simulink model "ModelGridFormingController"  (R2025b)
settings: Solver=ode1be  StartTime=0.0  StopTime=6  FixedStep=gridInverter.vsm.samplingTime  MaxStep=gridInverter.vsm.samplingTime  RelTol=1e-3  AbsTol=1e-3
PreLoadFcn:
  | % Parameterize the model
  | TestGridFormingControllerInputParameters;
values from neighbouring files (symbols this model uses):
  localSolverSampleTime = 100e-6    (= 0.0001)    [TestGridFormingControllerInputParameters.m]
undefined symbols (not defined in the file or in its folder): base, gridInverter
libraries: ee_lib x8, nesl_utility x5, fl_lib x3, eeGeneralControl x2, eeSinGeneratorThreePhase x1, GFMLibrary x1
CloseFcn:
  | try, close( 'GridFormingConverterNormalOperation'), end
  | try, close( 'GridFormingConverterActivePowerChange'), end
  | try, close( 'GridFormingConverterReactivePowerChange'), end
  | try, close( 'GridFormingConverterGridVoltageChange'), end
  | try, close( 'GridFormingConverterLocalLoadChange'), end
  | try, close( 'GridFormingConverterSmallGridFreqChange'), end
  | try, close( 'GridFormingConverterLargeGridFreqChange'), end
  | try, close( 'GridFormingConverterFullGridFreqChange'), end
  | try, close( 'GridFormingConverter10DegGridPhaseChange'), end
  | try, close( 'GridFormingConverter60DegGridPhaseChange'), end
  | try, close( 'GridFormingConverterPermanentFault'), end
  | try, close( 'GridFormingConverterTemporaryFault'), end
  | try, close( 'GridFormingConverterActivePowerChangeWithRipple'), end
  | try, close( 'GridFormingConverterIslanding'), end
  | try, close( 'GridFormingConverterDampingEffect'), end
  | try, close( 'GridFormingConverterIntertiaEffect'), end
  | try, close('GridFormingConverterVdControllerBodePlot'), end
  | try, close('GridFormingConverterControllerBodePlot'), end
  | try, close( 'GridFormingConverterThreePhaseFault'), end
  | try, close( 'GridFormingConverterThreePhaseFaultStandard'), end
  | try, close( 'GridFormingConverterCompareFaultRideMethod'), end
  | clear base currentLimitMethodSelected expectedSCR
  | clear grid gridInverter primaryBaseImpedance
  | clear realPowerMethodSelected scrSelected scrFactor
  | clear seconadryBaseImpedance shortCircuit
  | clear simulationTime systemSCR testConditionSelected
  | clear testCondition tout transformer TransmissionLine
  | clear gridVoltageProfileVal gridVoltageProfileTime
  | clear gridFrequencyProfileVal gridFrequencyProfileTime
  | clear gridVoltageProfileVal gridVoltageProfileTime
  | clear gridFrequencyProfileVal gridFrequencyProfileTime
  | clear gridPhaseProfileVal gridPhaseProfileTime
  | clear gfmRealPowerRefProfileVal gfmRealPowerRefProfileTime
  | clear gfmControllerRippleInjectMagVal gfmControllerRippleInjectMagTime
  | clear gfmControllerRippleInjectFreqVal gfmControllerRippleInjectFreqTime
  | clear gfmReactivePowerRefProfileVal gfmReactivePowerRefProfileTime
  | clear localLoadRealProfileVal localLoadRealProfileTime
  | clear localLoadReactiveProfileVal localLoadReactiveProfileTime
  | clear faultTriggerVal faultTriggerTime
  | clear circuitBreakerTripSignalVal circuitBreakerTripSignalTime
  | clear disturbanceTime realPartImpedance  localSolverSampleTime
  | clear SimlogGridFormingConverter temprySampleData
  | clear outValue outputTable plotFlag margintable testOutcome
  | clear realPart  XbyRtempFactor scrFactorXg scrFactorRg scrOut XbyROut systemSCR
  | clear outTable marginTable controllerName dampingArray inertiaConstantArray
  | clear imaginaryPart LogsoutGridFormingConverter faultImpedanceArray
  | clear outData
Description:
  | Design and Analysis of Grid-Forming Converter
settings Model: ExtModeTrigDuration=100  Creator=The MathWorks, Inc.  LastModifiedBy=vsolaise
settings SolverCC: AutoScaleAbsTol=off  AlgebraicLoopSolver=TrustRegion
settings DataIOCC: SaveOutput=off  DSMLogging=off  StateSaveName=tmp_raccel_xout  SignalLoggingName=LogsoutGridFormingConverter  OutputTimes=[0:1.1*3*Voc/(1*2000):1.1*3*Voc/1]  ReturnWorkspaceOutputsName=outData
settings OptimizationCC: ReuseModelBlockBuffer=off  EfficientMapNaN2IntZero=off
settings DebuggingCC: AlgebraicLoopMsg=none  StateNameClashWarn=warning  ArithmeticOperatorsInVariantConditions=warning
settings HardwareCC: ProdBitPerPointer=32.0  ProdBitPerSizeT=32.0  ProdBitPerPtrDiffT=32.0  ProdWordSize=32.0  ProdHWDeviceType=Intel->x86-32 (Windows32)  TargetBitPerPointer=64.0  TargetBitPerSizeT=64.0  TargetBitPerPtrDiffT=64.0  TargetLongLongMode=on  TargetIntDivRoundTo=Zero  TargetEndianess=LittleEndian  TargetWordSize=64.0  TargetHWDeviceType=MATLAB Host  ProdEqTarget=off
settings ModelReferenceCC: EnableRefExpFcnMdlSchedulingChecks=on  PropagateSignalLabelsOutOfModel=off
settings SFSimCC: CustomCodeUndefinedFunction=UseInterfaceOnly
settings RTWCC: SystemTargetFile=raccel.tlc  TemplateMakefile=raccel_default_tmf  RTWVerbose=off  RTWUseSimCustomCode=on  GPUComputeCapability=3.5
settings CodeAppCC: GenerateComments=off  MaxIdLength=128.0  SimulinkBlockComments=off
settings RaccelTargetCC: ExtModeTransport=0.0  ExtModeStaticAllocSize=1000000.0  ENABLE_SLEXEC_SSBRIDGE=1.0  RTWCAPIParams=on  RTWCAPIRootIO=on  TargetLangStandard=C99 (ISO)  MultiwordLength=2048.0  DynamicStringBufferSize=256.0  PreserveMATLABNamespacesInGeneratedCode=on  SubcomponentCodeInterfacePackaging=Reusable function  InstructionSetFMA=off  OptimizeReductions=off  LogToMDFFile=off
settings SimscapeCC: SimscapeLogType=all  SimscapeLogSimulationStatistics=on  SimscapeLogName=SimlogGridFormingConverter  SimscapeLogLimitData=off

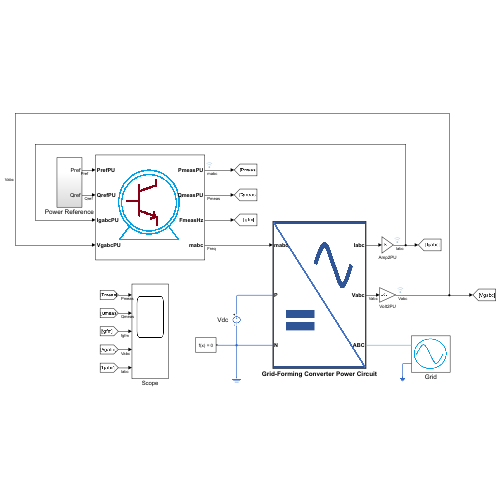
[thumbnail: Simulink's stored preview of the top-level diagram]
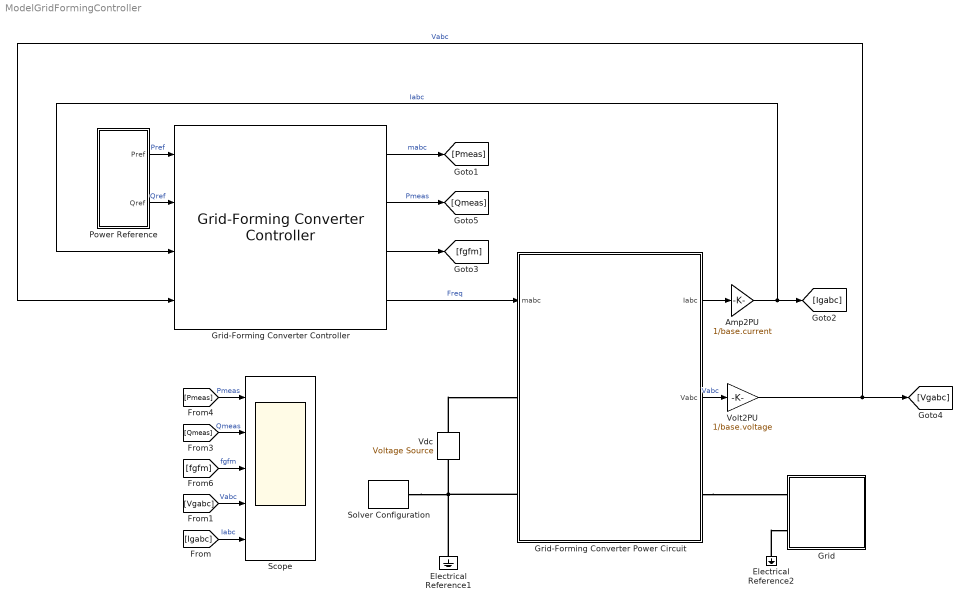
== system ModelGridFormingController ==
  Amp2PU : Gain  Gain=1/base.current
  Electrical Reference1 : fl_lib/Electrical/Electrical Elements/Electrical Reference
  Electrical Reference2 : fl_lib/Electrical/Electrical Elements/Electrical Reference
  Grid : Subsystem
      mask Display: image('$imagefile'); % Use "Edit Image" on toolstrip to change.
  Grid-Forming Converter Controller : GFMLibrary/Grid-Forming Converter Controller  power=500e3  gridLineVoltage=415  powerFreq=50  dcBusVoltage=1100  measSampleTime=0.0001  powerControl=Virtual Synchronous Machine  activePowerSampleTime=0.0001  droopSlope=0.01  droopT1=0.005  droopT2=0.006  droopTC=0.015  vsmPmeasFilterTC=0.001  vsmFreqDroop=10  vsmInertiaTC=1  vsmDampingConst=1.056  dampingPowerMaxLimit=0.7  dampingPowerMinLimit=-0.6  freqMeasTimeConst=0.15  freqOption=Grid Frequency Measurement  voltreference=1  QVoltFilterTC=0.001  QVoltDroop=0.3  lowVoltageSupportGain=1.5  currentLimit=Virtual Impedance  maxSatCurrentLimit=1.4  maxVICurrentLimit=1.2  ctLimitVirtualImp=0.20625  ctLimitXbyR=13.2  ctLimitDelayTime=0.001  currentSatTime=0.001  currentVITimeConst=0.001  modeTransferTime=10*gridInverter.controller.CurrentControlSampleTime  voltControlTs=0.0001  vdPGain=0.3  VdIGain=180  VdMaxCt=1.8  VdMinCt=-1.8  VqPGain=0.3  VqIGain=180  VqMaxCt=1.8  VqMinCt=-1.8  vdvqLPFTimeConst=0.005  currentControlTs=0.0001  filterInductance=0.00010964  IdPGain=1.5  IdIGain=10  IqPGain=1.5  IqIGain=10
  Grid-Forming Converter Power Circuit : Subsystem
      mask Display: image('$imagefile'); % Use "Edit Image" on toolstrip to change.
  Power Reference : Subsystem
  Scope : Scope  NumInputPorts=5
      settings: Title=Active Power Measured in pu  ActiveDisplayYMinimum=-0.18492062532329751  ActiveDisplayYMaximum=1.0233144736966111
  Solver Configuration : nesl_utility/Solver Configuration  PhysicalDomain=network_engine_domain  SubClassName=solver  LeftPortType=input  RightPortType=generic  Tones=[]  Harmonics=[]  SimulateNoise=off  Profile=off  UseLocalSampling=off  EnableSwitchedLinearOptims=on  FrequencyDomain=off  UseCCode=off  RelTol=0.001  AbsTol=1e-06  MinStep=1e-09  ToWorkspace=off  RevertToSquareIcSolve=off  NumHomotopyIterations=100  PhasorMode=off  PhasorModeNumHarmonics=1  ConsistencySolver=NEWTON_FTOL  IndexReductionMethod=DerivativeReplacement  DoDC=off  ResidualTolerance=1e-09  ConsistencyTolSource=GLOBAL  ConsistencyAbsTol=0.001  ConsistencyRelTol=0.001  ConsistencyTolFactor=0.001  UseLocalSolver=on  LocalSolverChoice=NE_BACKWARD_EULER_ADVANCER  ResolveIndetEquations=on  FunctionEvalNumThread=1  LocalSolverSampleTime=100e-6  DoFixedCost=on  MaxNonlinIter=3  MaxModeIter=2  ComputeImpulses=off  ImpulseIterations=2  LinearAlgebra=auto  LinearAlgebraNumThread=0  EquationFormulation=NE_TIME_EF  DelaysMemoryBudget=1024  AutomaticFiltering=on  FilteringTimeConstant=0.001  PartitionStorageMethod=AS_NEEDED  PartitionMemoryBudget=1024  PartitionMethod=ROBUST  MultibodyUseLocalSolver=off  MultibodyLocalSolverChoice=ODE1  MultibodyLocalSolverSampleTime=0.001
  Vdc : ee_lib/Sources/Voltage Source  dc_voltage=gridInverter.DCVoltage V  ac_voltage=0 V  ac_shift=0 rad  ac_frequency=0 Hz  noise_mode=ee.enum.sources.noise.Disabled  PSD=0 V^2/Hz  sample_time=1e-3 s  repeatability=ee.enum.sources.repeatability.NotRepeatable  user_seed=0  auto_seed=3499211588  i_specify=off  i_priority=None  i=0 A  i_nominal_specify=off  i_nominal_value=1  i_nominal_unit=A  v_specify=off  v_priority=None  v=0 V  v_nominal_specify=off  v_nominal_value=1  v_nominal_unit=V
  Volt2PU : Gain  Gain=1/base.voltage
  wires:
  [Pmeas] -> Scope/1  "Pmeas"
  [Qmeas] -> Scope/2  "Qmeas"
  [fgfm] -> Scope/3  "fgfm"
  [Vgabc] -> Scope/4  "Vabc"
  [Igabc] -> Scope/5  "Iabc"
  Power Reference/1(Pref) -> Grid-Forming Converter Controller/1  "Pref"
  Power Reference/2(Qref) -> Grid-Forming Converter Controller/2  "Qref"
  Grid-Forming Converter Controller/3 -> [fgfm]
  Grid-Forming Converter Power Circuit/1(Iabc) -> Amp2PU/1
  Volt2PU/1 -> Grid-Forming Converter Controller/4, [Vgabc]  "Vabc"
  Grid-Forming Converter Power Circuit/2(Vabc) -> Volt2PU/1  "Vabc"
  Amp2PU/1 -> Grid-Forming Converter Controller/3, [Igabc]  "Iabc"
  Grid-Forming Converter Controller/4 -> Grid-Forming Converter Power Circuit/1(mabc)  "Freq"
  Grid-Forming Converter Controller/2 -> [Qmeas]  "Pmeas"
  Grid-Forming Converter Controller/1 -> [Pmeas]  "mabc"
  connections:
  Electrical Reference2/LConn1 -- Grid/LConn2
  Vdc/LConn1 -- Grid-Forming Converter Power Circuit/LConn1
  Grid-Forming Converter Power Circuit/LConn2 -- Solver Configuration/RConn1 -- Electrical Reference1/LConn1 -- Vdc/RConn1
  Grid-Forming Converter Power Circuit/RConn1 -- Grid/LConn1

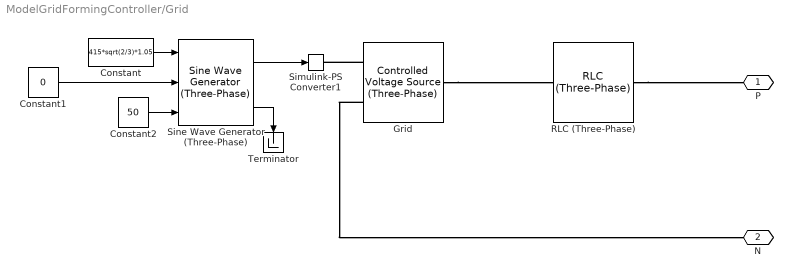
== system ModelGridFormingController/Grid ==
  Constant : Constant  Value=415*sqrt(2/3)*1.05
  Constant1 : Constant  Value=0
  Constant2 : Constant  Value=50
  Grid : ee_lib/Sources/Controlled Voltage Source (Three-Phase)  input_option=ee.enum.inputType.instantaneous  FRated=60 Hz
      settings: InternalSimscapePortConfiguration="{\"Bottom\":[],\"Left\":[{\"id\":\"S\",\"label\":\"S\",\"type\":\"input\"},{\"id\":\"n\",\"label\":\"n\",\"type\":\"foundation.electrical.electrical\"}],\"Right\":[{\"id\":\"N\",\"label\":\"~\",\"type\":\"foundation.electrical.three_phase\"}],\"Top\":[]}"
  RLC (Three-Phase) : ee_lib/Passive/RLC Assemblies/RLC (Three-Phase)  port_option=ee.enum.threePhasePort.composite  component_structure=ee.enum.rlc.structure.R  R=0.1 Ohm  L=1e-3 H  C=1e-6 F  R_parasitic=0 Ohm  G_parasitic=0 1/Ohm  IL_specify=off  IL_priority=High  IL=[0, 0, 0] A  IL_nominal_specify=off  IL_nominal_value=1  IL_nominal_unit=A  VC_specify=off  VC_priority=High  VC=[0, 0, 0] V  VC_nominal_specify=off  VC_nominal_value=1  VC_nominal_unit=V
      settings: InternalSimscapePortConfiguration="{\"Bottom\":[],\"Left\":[{\"id\":\"N1\",\"label\":\"~1\",\"type\":\"foundation.electrical.three_phase\"}],\"Right\":[{\"id\":\"N2\",\"label\":\"~2\",\"type\":\"foundation.electrical.three_phase\"}],\"Top\":[]}"
  Simulink-PS Converter1 : nesl_utility/Simulink-PS Converter  PhysicalDomain=network_engine_domain  SubClassName=ps_input  LeftPortType=input  RightPortType=output  PseudoPeriodic=off  Frequencies=[]  NoiseDistribution=none  NoiseParameters=[]  Unit=1  AffineConversion=off  FilteringAndDerivatives=provide  SimscapeFilterOrder=1  InputFilterTimeConstant=0.001  UdotUserProvided=0
  Sine Wave Generator (Three-Phase) : eeSinGeneratorThreePhase/Sine Wave Generator (Three-Phase)  Ts=100e-6
  Terminator : Terminator
  P : PMIOPort  Side=Left
  N : PMIOPort  Port=2  Side=Left
  wires:
  Sine Wave Generator (Three-Phase)/1 -> Simulink-PS Converter1/1
  Sine Wave Generator (Three-Phase)/2 -> Terminator/1
  Constant2/1 -> Sine Wave Generator (Three-Phase)/3
  Constant1/1 -> Sine Wave Generator (Three-Phase)/2
  Constant/1 -> Sine Wave Generator (Three-Phase)/1
  connections:
  Grid/LConn1 -- Simulink-PS Converter1/RConn1
  Grid/LConn2 -- N/RConn1
  Grid/RConn1 -- RLC (Three-Phase)/LConn1
  RLC (Three-Phase)/RConn1 -- P/RConn1

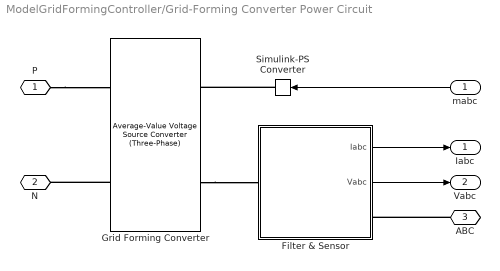
== system ModelGridFormingController/Grid-Forming Converter Power Circuit ==
  mabc : Inport
  Filter & Sensor : Subsystem
      mask Display: image('$imagefile'); % Use "Edit Image" on toolstrip to change.
  Grid Forming Converter : ee_lib/Semiconductors & Converters/Converters/Average-Value Voltage Source Converter (Three-Phase)  port_option=ee.enum.threePhasePort.composite  frequency_option=ee.enum.converters.frequency.variable  input_option=ee.enum.converters.inputOption.ModWave  FRated=50 Hz  losses_parameterization=ee.enum.converters.losses.fixed  Pfixed=10 W  ks=0.01  kc1=1.7 V  kc2=0.01 Ohm  Ploss_vect=[100, 800, 1870, 3250, 4900] W  Irms_vect=[10, 100, 200, 300, 400] A  Vdc_nom=300 V  thermal_mass=30000 J/K  temperature_specify=off  temperature_priority=High  temperature=298.15 K  temperature_nominal_specify=off  temperature_nominal_value=1  temperature_nominal_unit=K
      settings: InternalSimscapePortConfiguration="{\"Bottom\":[],\"Left\":[{\"id\":\"ModWave\",\"label\":\"ModWave\",\"type\":\"input\"},{\"id\":\"N\",\"label\":\"~\",\"type\":\"foundation.electrical.three_phase\"}],\"Right\":[{\"id\":\"p\",\"label\":\"+\",\"type\":\"foundation.electrical.electrical\"},{\"id\":\"n\",\"label\":\"-\",\"type\":\"foundation.electrical.electrical\"}],\"Top\":[]}"
  Simulink-PS Converter : nesl_utility/Simulink-PS Converter  PhysicalDomain=network_engine_domain  SubClassName=ps_input  LeftPortType=input  RightPortType=output  PseudoPeriodic=off  Frequencies=[]  NoiseDistribution=none  NoiseParameters=[]  Unit=1  AffineConversion=off  FilteringAndDerivatives=provide  SimscapeFilterOrder=1  InputFilterTimeConstant=0.001  UdotUserProvided=0
  P : PMIOPort  Side=Left
  N : PMIOPort  Port=2  Side=Left
  ABC : PMIOPort  Port=3  Side=Right
  Iabc : Outport
  Vabc : Outport  Port=2
  wires:
  mabc/1 -> Simulink-PS Converter/1
  Filter & Sensor/1(Iabc) -> Iabc/1
  Filter & Sensor/2(Vabc) -> Vabc/1
  connections:
  Grid Forming Converter/LConn2 -- Filter & Sensor/LConn1
  Simulink-PS Converter/RConn1 -- Grid Forming Converter/LConn1
  P/RConn1 -- Grid Forming Converter/RConn1
  ABC/RConn1 -- Filter & Sensor/RConn1
  Grid Forming Converter/RConn2 -- N/RConn1

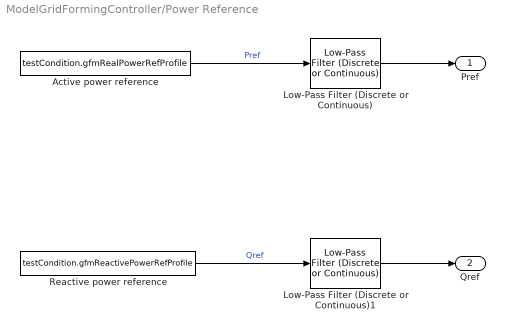
== system ModelGridFormingController/Power Reference ==
  Active power reference : FromWorkspace  VariableName=testCondition.gfmRealPowerRefProfile  SampleTime=localSolverSampleTime  OutputAfterFinalValue=Holding final value
  Low-Pass Filter (Discrete or Continuous) : eeGeneralControl/Low-Pass Filter (Discrete or Continuous)  K=1  T=5e-2  B=inf  A=-inf  init_option=Inherited from block input  x0=0  Ts=-1
  Low-Pass Filter (Discrete or Continuous)1 : eeGeneralControl/Low-Pass Filter (Discrete or Continuous)  K=1  T=5e-2  B=inf  A=-inf  init_option=Inherited from block input  x0=0  Ts=-1
  Reactive power reference : FromWorkspace  VariableName=testCondition.gfmReactivePowerRefProfile  SampleTime=localSolverSampleTime  OutputAfterFinalValue=Holding final value
  Pref : Outport
  Qref : Outport  Port=2
  wires:
  Active power reference/1 -> Low-Pass Filter (Discrete or Continuous)/1  "Pref"
  Reactive power reference/1 -> Low-Pass Filter (Discrete or Continuous)1/1  "Qref"
  Low-Pass Filter (Discrete or Continuous)/1 -> Pref/1
  Low-Pass Filter (Discrete or Continuous)1/1 -> Qref/1

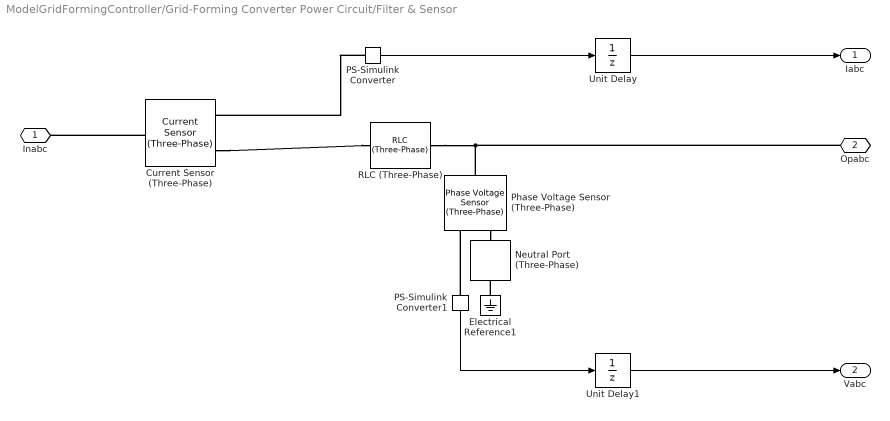
== system ModelGridFormingController/Grid-Forming Converter Power Circuit/Filter & Sensor ==
  Current Sensor (Three-Phase) : ee_lib/Sensors & Transducers/Current Sensor (Three-Phase)
  Electrical Reference1 : fl_lib/Electrical/Electrical Elements/Electrical Reference
  Neutral Port (Three-Phase) : ee_lib/Connectors & References/Neutral Port (Three-Phase)  G_parasitic=1e-12 1/Ohm
      settings: InternalSimscapePortConfiguration="{\"Bottom\":[],\"Left\":[{\"id\":\"N\",\"label\":\"~\",\"type\":\"foundation.electrical.three_phase\"}],\"Right\":[{\"id\":\"n\",\"label\":\"n\",\"type\":\"foundation.electrical.electrical\"}],\"Top\":[]}"
  PS-Simulink Converter : nesl_utility/PS-Simulink Converter  PhysicalDomain=network_engine_domain  SubClassName=ps_output  LeftPortType=input  RightPortType=output  PseudoPeriodic=off  Frequencies=[]  VectorFormat=inherit  Unit=inherit  AffineConversion=off
  PS-Simulink Converter1 : nesl_utility/PS-Simulink Converter  PhysicalDomain=network_engine_domain  SubClassName=ps_output  LeftPortType=input  RightPortType=output  PseudoPeriodic=off  Frequencies=[]  VectorFormat=inherit  Unit=inherit  AffineConversion=off
  Phase Voltage Sensor (Three-Phase) : ee_lib/Sensors & Transducers/Phase Voltage Sensor (Three-Phase)
  RLC (Three-Phase) : ee_lib/Passive/RLC Assemblies/RLC (Three-Phase)  port_option=ee.enum.threePhasePort.composite  component_structure=ee.enum.rlc.structure.SeriesRL  R=gridInverter.lineResistance Ohm  L=gridInverter.L H  C=1e-6 F  R_parasitic=0 Ohm  G_parasitic=0 1/Ohm  IL_specify=off  IL_priority=High  IL=[0, 0, 0] A  IL_nominal_specify=off  IL_nominal_value=1  IL_nominal_unit=A  VC_specify=off  VC_priority=High  VC=[0, 0, 0] V  VC_nominal_specify=off  VC_nominal_value=1  VC_nominal_unit=V
      settings: InternalSimscapePortConfiguration="{\"Bottom\":[],\"Left\":[{\"id\":\"N1\",\"label\":\"~1\",\"type\":\"foundation.electrical.three_phase\"}],\"Right\":[{\"id\":\"N2\",\"label\":\"~2\",\"type\":\"foundation.electrical.three_phase\"}],\"Top\":[]}"
  Unit Delay : UnitDelay  SampleTime=-1  HasFrameUpgradeWarning=on
  Unit Delay1 : UnitDelay  SampleTime=-1  HasFrameUpgradeWarning=on
  Inabc : PMIOPort  Side=Left
  Opabc : PMIOPort  Port=2  Side=Right
  Iabc : Outport
  Vabc : Outport  Port=2
  wires:
  PS-Simulink Converter1/1 -> Unit Delay1/1
  Unit Delay/1 -> Iabc/1
  PS-Simulink Converter/1 -> Unit Delay/1
  Unit Delay1/1 -> Vabc/1
  connections:
  PS-Simulink Converter1/LConn1 -- Phase Voltage Sensor (Three-Phase)/RConn1
  Current Sensor (Three-Phase)/RConn2 -- RLC (Three-Phase)/LConn1
  Current Sensor (Three-Phase)/LConn1 -- Inabc/RConn1
  PS-Simulink Converter/LConn1 -- Current Sensor (Three-Phase)/RConn1
  Phase Voltage Sensor (Three-Phase)/LConn1 -- Opabc/RConn1 -- RLC (Three-Phase)/RConn1
  Phase Voltage Sensor (Three-Phase)/RConn2 -- Neutral Port (Three-Phase)/LConn1
  Electrical Reference1/LConn1 -- Neutral Port (Three-Phase)/RConn1
